simulink model "odev5_tekrar_iremelmas_kara"  (R2023b)
settings: Solver=ode23tb  StartTime=0.0  StopTime=0.1  RelTol=1e-3
libraries: spsCurrentMeasurementLib x18, spsSeriesRLCBranchLib x15, spsMeanLib x9, spsDiodeLib x6, spsMosfetLib x6, spsVoltageMeasurementLib x6, spsDCVoltageSourceLib x3, spsGroundLib x3, spsLinearTransformerLib x3, spsTHDLib x3, spspowerguiLib x1
settings Model: Creator=ireme  LastModifiedBy=ireme

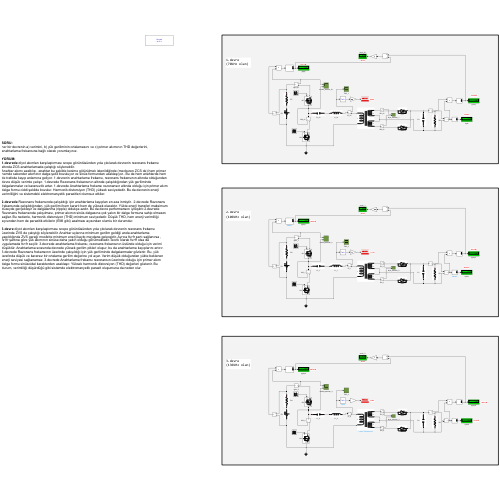
[thumbnail: Simulink's stored preview of the top-level diagram]
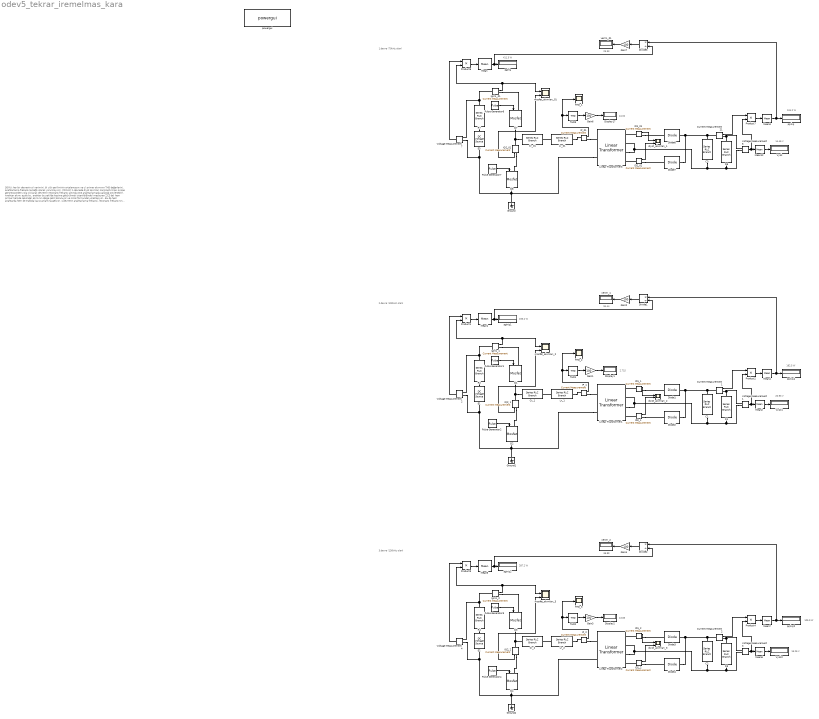
== system odev5_tekrar_iremelmas_kara ==
  note: 1.devre
      | (70kHz olan)
  note: 14.46 V
  note: 2.devre
      | (100kHz olan)
  note: 20.93 V
  note: 3.devre
      | (130kHz olan)
  note: 15.26 V
  note: 104.2 W
  note: 411.3 W
  note: 25.33
  note: 24.02
  note: 182.5 W
  note: 2.715
  note: 94.44
  note: 193.2 W
  note: 105.9 W
  note: 36.89
  note: 13.83
  note: 287.2 W
  note: SORU:
      | her bir devrenin a) verimini, b) yük geriliminin ortalamasını ve c) primer akımının THD değerlerini, anahtarlama frekansına bağlı olarak yorumlayınız.
      |
      | YORUM:
      | 1.devrede diyot akımları karşılaştırması scope görüntüsünden yola çıkılarak devrenin rezonans frekansı altında ZCS anahtarlamada çalıştığı söylenebilir.
      | Anahtar akımı azaltılıp , anahtar bu şekilde kesime götürülmek istenildiğinde (mecburen ZCS de) hem primer hemde sekonder akımının dalga şekli bozuluyor ve sinüs formundan uzaklaşıyor.. Bu da hem anahtarda hem de trafoda kayıp anlamına geliyor. 1.devrenin anahtarlama frekansı, rezonans frekansının altında olduğundan devre düşük verimle çalışır. 1.devrede Rezonans frekansının altında çalışıldığından yük geriliminde dalgalanmalar ve kararsızlık artar. 1.devrede Anahtarlama frekansı rezonansın altında olduğu için primer akım dalga formu ciddi şekilde bozulur. Harmonik distorsiyon (THD) yüksek seviyededir. Bu da devrenin enerji verimliliğini ve sistemdeki elektromanyetik parazitleri olumsuz etkiler.
      |
      | 2.devrede Rezonans frekansında çalışıldığı için anahtarlama kayıpları en aza inmiştir. 2.devrede Rezonans frekansında çalışıldığından, yük gerilimi hem kararlı hem de yüksek olacaktır. Yükte enerji transferi maksimum düzeyde gerçekleşir ve dalgalanma (ripple) oldukça azdır. Bu da devre performansını iyileştirir. 2.devrede Rezonans frekansında çalışılması, primer akımın sinüs dalgasına çok yakın bir dalga formuna sahip olmasını sağlar. Bu nedenle, harmonik distorsiyon (THD) minimum seviyededir. Düşük THD, hem enerji verimliliği açısından hem de parazitik etkilerin (EMI gibi) azalması açısından olumlu bir durumdur.
      |
      | 3.devre diyot akımları karşılaştırması scope görüntüsünden yola çıkılarak devrenin rezonans frekansı üzerinde ZVS de çalıştığı söylenebilir. Anahtar uçlarına minimum gerilim geldiği anda anahtarlama yapıldığında ZVS gereği mosfette minimum enerji kaybı meydana gelecektir. Ayrıca fs>fr şartı sağlanırsa , fs<fr şartına göre yük akımının sinüse daha yakın olduğu görülmektedir.Teorik olarak fs>fr olsa da uygulamada fs<fr seçilir. 3.devrede anahtarlama frekansı, rezonans frekansının üstünde olduğu için verimi düşüktür. Anahtarlama sırasında devrede yüksek gerilim pikleri oluşur, bu da anahtarlama kayıplarını artırır. 3.devrede Rezonans frekansının üzerinde çalışıldığı için yük geriliminde dalgalanmalar gözlenir. Bu, yük tarafında düşük ve kararsız bir ortalama gerilim değerine yol açar. Verim düşük olduğundan yükte beklenen enerji seviyesi sağlanamaz. 3.devrede Anahtarlama frekansı rezonansın üzerinde olduğu için primer akım dalga formu sinüsoidal karakterden uzaklaşır. Yüksek harmonik distorsiyon (THD) değerleri gözlenir. Bu durum, verimliliği düşürdüğü gibi sistemde elektromanyetik parazit oluşumuna da neden olur.
  C1 : spsSeriesRLCBranchLib/Series RLC Branch  LConnTagsString=__new0  RConnTagsString=__new0  BranchType=C  Resistance=1  Inductance=1e-3  SetiL0=off  InitialCurrent=0  Capacitance=150e-3  Setx0=off  InitialVoltage=0  Measurements=None
  C2 : spsSeriesRLCBranchLib/Series RLC Branch  LConnTagsString=__new0  RConnTagsString=__new0  BranchType=C  Resistance=1  Inductance=1e-3  SetiL0=off  InitialCurrent=0  Capacitance=150e-3  Setx0=off  InitialVoltage=0  Measurements=None
  C3 : spsSeriesRLCBranchLib/Series RLC Branch  LConnTagsString=__new0  RConnTagsString=__new0  BranchType=C  Resistance=1  Inductance=1e-3  SetiL0=off  InitialCurrent=0  Capacitance=150e-3  Setx0=off  InitialVoltage=0  Measurements=None
  Cr_01 : spsSeriesRLCBranchLib/Series RLC Branch  LConnTagsString=__new0  RConnTagsString=__new0  BranchType=C  Resistance=1  Inductance=1e-3  SetiL0=off  InitialCurrent=0  Capacitance=22e-9  Setx0=off  InitialVoltage=0  Measurements=None
  Cr_1 : spsSeriesRLCBranchLib/Series RLC Branch  LConnTagsString=__new0  RConnTagsString=__new0  BranchType=C  Resistance=1  Inductance=1e-3  SetiL0=off  InitialCurrent=0  Capacitance=22e-9  Setx0=off  InitialVoltage=0  Measurements=None
  Cr_2 : spsSeriesRLCBranchLib/Series RLC Branch  LConnTagsString=__new0  RConnTagsString=__new0  BranchType=C  Resistance=1  Inductance=1e-3  SetiL0=off  InitialCurrent=0  Capacitance=22e-9  Setx0=off  InitialVoltage=0  Measurements=None
  Current Measurement1 : spsCurrentMeasurementLib/Current Measurement  PhasorSimulation=off  OutputType=Complex  PSBequivalent=0
  Current Measurement2 : spsCurrentMeasurementLib/Current Measurement  PhasorSimulation=off  OutputType=Complex  PSBequivalent=0
  Current Measurement21 : spsCurrentMeasurementLib/Current Measurement  PhasorSimulation=off  OutputType=Complex  PSBequivalent=0
  Diode{1..4,6..7} (6 alike) : spsDiodeLib/Diode  Ron=0.001  Lon=0  Vf=0.8  IC=0  UseSnubber=0  Rs=500  Cs=250e-9  Measurements=off
  Display1 : Display
  Display17 : Display
  Display2 : Display
  Divide1 : Product  Inputs=*/
  Divide2 : Product  Inputs=*/
  Divide3 : Product  Inputs=*/
  E1 : spsDCVoltageSourceLib/DC Voltage Source  Amplitude=390  Measurements=None
  E2 : spsDCVoltageSourceLib/DC Voltage Source  Amplitude=390  Measurements=None
  E3 : spsDCVoltageSourceLib/DC Voltage Source  Amplitude=390  Measurements=None
  Gain{1..4,6..7} (6 alike) : Gain  Gain=100
  Ground : spsGroundLib/Ground  LConnTagsString=a
  Ground1 : spsGroundLib/Ground  LConnTagsString=a
  Ground2 : spsGroundLib/Ground  LConnTagsString=a
  ID1_01 : spsCurrentMeasurementLib/Current Measurement  PhasorSimulation=off  OutputType=Complex  PSBequivalent=0
  ID1_1 : spsCurrentMeasurementLib/Current Measurement  PhasorSimulation=off  OutputType=Complex  PSBequivalent=0
  ID1_2 : spsCurrentMeasurementLib/Current Measurement  PhasorSimulation=off  OutputType=Complex  PSBequivalent=0
  ID2_01 : spsCurrentMeasurementLib/Current Measurement  PhasorSimulation=off  OutputType=Complex  PSBequivalent=0
  ID2_1 : spsCurrentMeasurementLib/Current Measurement  PhasorSimulation=off  OutputType=Complex  PSBequivalent=0
  ID2_2 : spsCurrentMeasurementLib/Current Measurement  PhasorSimulation=off  OutputType=Complex  PSBequivalent=0
  IP_01 : spsCurrentMeasurementLib/Current Measurement  PhasorSimulation=off  OutputType=Complex  PSBequivalent=0
  IP_1 : spsCurrentMeasurementLib/Current Measurement  PhasorSimulation=off  OutputType=Complex  PSBequivalent=0
  IP_2 : spsCurrentMeasurementLib/Current Measurement  PhasorSimulation=off  OutputType=Complex  PSBequivalent=0
  IQ2_01 : spsCurrentMeasurementLib/Current Measurement  PhasorSimulation=off  OutputType=Complex  PSBequivalent=0
  IQ2_1 : spsCurrentMeasurementLib/Current Measurement  PhasorSimulation=off  OutputType=Complex  PSBequivalent=0
  IQ2_2 : spsCurrentMeasurementLib/Current Measurement  PhasorSimulation=off  OutputType=Complex  PSBequivalent=0
  Igiris_01 : spsCurrentMeasurementLib/Current Measurement  PhasorSimulation=off  OutputType=Complex  PSBequivalent=0
  Igiris_1 : spsCurrentMeasurementLib/Current Measurement  PhasorSimulation=off  OutputType=Complex  PSBequivalent=0
  Igiris_2 : spsCurrentMeasurementLib/Current Measurement  PhasorSimulation=off  OutputType=Complex  PSBequivalent=0
  Linear Transformer1 : spsLinearTransformerLib/Linear Transformer  UNITS=SI  NominalPower=[ 300 150e3]  winding1=[36 0 0]  winding2=[4 0 0]  ThreeWindings=on  winding3=[4 0 0]  RmLm=[1e6 565e-06]  Measurements=None  DataType=on
  Linear Transformer2 : spsLinearTransformerLib/Linear Transformer  UNITS=SI  NominalPower=[ 300 150e3]  winding1=[36 0 0]  winding2=[4 0 0]  ThreeWindings=on  winding3=[4 0 0]  RmLm=[1e6 565e-06]  Measurements=None  DataType=on
  Linear Transformer3 : spsLinearTransformerLib/Linear Transformer  UNITS=SI  NominalPower=[ 300 150e3]  winding1=[36 0 0]  winding2=[4 0 0]  ThreeWindings=on  winding3=[4 0 0]  RmLm=[1e6 565e-06]  Measurements=None  DataType=on
  Lr_01 : spsSeriesRLCBranchLib/Series RLC Branch  LConnTagsString=__new0  RConnTagsString=__new0  BranchType=L  Resistance=1  Inductance=113e-6  SetiL0=off  InitialCurrent=0  Capacitance=1e-6  Setx0=off  InitialVoltage=0  Measurements=None
  Lr_1 : spsSeriesRLCBranchLib/Series RLC Branch  LConnTagsString=__new0  RConnTagsString=__new0  BranchType=L  Resistance=1  Inductance=113e-6  SetiL0=off  InitialCurrent=0  Capacitance=1e-6  Setx0=off  InitialVoltage=0  Measurements=None
  Lr_2 : spsSeriesRLCBranchLib/Series RLC Branch  LConnTagsString=__new0  RConnTagsString=__new0  BranchType=L  Resistance=1  Inductance=113e-6  SetiL0=off  InitialCurrent=0  Capacitance=1e-6  Setx0=off  InitialVoltage=0  Measurements=None
  Mean{,1..2,5..6,12} (6 alike) : spsMeanLib/Mean  Freq=50  Vinit=0  Ts=0
  Mean3 : spsMeanLib/Mean  Freq=70e3  Vinit=0  Ts=0
  Mean4 : spsMeanLib/Mean  Freq=100e3  Vinit=0  Ts=0
  Mean7 : spsMeanLib/Mean  Freq=130e3  Vinit=0  Ts=0
  Product{1..4,6..7} (6 alike) : Product
  Pulse Generator1 : DiscretePulseGenerator  PulseType=Time based  Period=1/(100e3)  PulseWidth=50
  Pulse Generator2 : DiscretePulseGenerator  PulseType=Time based  Period=1/(100e3)  PulseWidth=50  PhaseDelay=1/(2*100e3)
  Pulse Generator3 : DiscretePulseGenerator  PulseType=Time based  Period=1/(130e3)  PulseWidth=50
  Pulse Generator4 : DiscretePulseGenerator  PulseType=Time based  Period=1/(130e3)  PulseWidth=50  PhaseDelay=1/(2*130e3)
  Pulse Generator6 : DiscretePulseGenerator  PulseType=Time based  Period=1/(70e3)  PulseWidth=50
  Pulse Generator7 : DiscretePulseGenerator  PulseType=Time based  Period=1/(70e3)  PulseWidth=50  PhaseDelay=1/(2*70e3)
  Q{1..4,7..8} (6 alike) : spsMosfetLib/Mosfet  Ron=0.1  Lon=0  Rd=0.01  Vfd=0  IC=0  Rs=1e5  Cs=inf  Measurements=off
  R1 : spsSeriesRLCBranchLib/Series RLC Branch  LConnTagsString=__new0  RConnTagsString=__new0  BranchType=R  Resistance=2.4  Inductance=1e-3  SetiL0=off  InitialCurrent=0  Capacitance=1e-6  Setx0=off  InitialVoltage=0  Measurements=None
  R2 : spsSeriesRLCBranchLib/Series RLC Branch  LConnTagsString=__new0  RConnTagsString=__new0  BranchType=R  Resistance=1e-6  Inductance=1e-3  SetiL0=off  InitialCurrent=0  Capacitance=1e-6  Setx0=off  InitialVoltage=0  Measurements=None
  R3 : spsSeriesRLCBranchLib/Series RLC Branch  LConnTagsString=__new0  RConnTagsString=__new0  BranchType=R  Resistance=2.4  Inductance=1e-3  SetiL0=off  InitialCurrent=0  Capacitance=1e-6  Setx0=off  InitialVoltage=0  Measurements=None
  R4 : spsSeriesRLCBranchLib/Series RLC Branch  LConnTagsString=__new0  RConnTagsString=__new0  BranchType=R  Resistance=1e-6  Inductance=1e-3  SetiL0=off  InitialCurrent=0  Capacitance=1e-6  Setx0=off  InitialVoltage=0  Measurements=None
  R6 : spsSeriesRLCBranchLib/Series RLC Branch  LConnTagsString=__new0  RConnTagsString=__new0  BranchType=R  Resistance=2.4  Inductance=1e-3  SetiL0=off  InitialCurrent=0  Capacitance=1e-6  Setx0=off  InitialVoltage=0  Measurements=None
  R7 : spsSeriesRLCBranchLib/Series RLC Branch  LConnTagsString=__new0  RConnTagsString=__new0  BranchType=R  Resistance=1e-6  Inductance=1e-3  SetiL0=off  InitialCurrent=0  Capacitance=1e-6  Setx0=off  InitialVoltage=0  Measurements=None
  THD1 : spsTHDLib/THD  Freq=100e3  Ts=0
  THD2 : spsTHDLib/THD  Freq=130e3  Ts=0
  THD3 : spsTHDLib/THD  Freq=70e3  Ts=0
  THD_1 : Scope
  THD_2 : Scope
  THD_3 : Scope
  Voltage Measurement{1..4,6..7} (6 alike) : spsVoltageMeasurementLib/Voltage Measurement  PhasorSimulation=off  OutputType=Complex  PSBequivalent=0
  Vyük : Display
  Vyük1 : Display
  Vyük2 : Display
  diyot_akımları_1 : Scope  NumInputPorts=2
  diyot_akımları_2 : Scope  NumInputPorts=2
  diyot_akımları_3 : Scope  NumInputPorts=2
  mosfet_akımları_01 : Scope  NumInputPorts=2
  mosfet_akımları_2 : Scope  NumInputPorts=2
  mosfet_akımları_3 : Scope  NumInputPorts=2
  pgiriş : Display
  pgiriş1 : Display
  pgiriş2 : Display
  powergui : spspowerguiLib/powergui  Priority=1  SimulationMode=Discrete  SampleTime=1e-7  frequency=60  Iterations=50  frequencyindice=0  Pbase=100e6  ErrMax=1e-4  UnitsV=kV  UnitsW=MW  buscounter=0  FunctionMessages=off  echomessages=off  EnableUseOfTLC=off  CurrentSourceSwitches=off  DisableSnubberDevices=off  DisableRonSwitches=off  DisableVfSwitches=off  DisplayEquations=off  AutomaticDiscreteSolvers=off  SolverType=Tustin/Backward Euler (TBE)  Interpol=off  ExternalGateDelay=off  methode=off  Ts=100  x0status=zero  SPID=on  SwTol=0  HookPort=off  NonlinearTolerance=1e-4  nMaxIteration=100  ContinueOnMaxIteration=off  RestoreLinks=warning  ResistiveCurrentMeasurement=off  Frange=[0:2:500]  Ylog=off  Xlog=on  ShowGrid=off  save=off  variable=ZData  structure=0  ZoomFFT=off  StartTime=0.0  cycles=1  DisplayStyle=1  fundamental=60  FreqAxis=off  MaxFrequency=1000  frequencyindicesteady=1  RmsSteady=1  display=off
  pçıkış : Display
  pçıkış1 : Display
  pçıkış2 : Display
  verim_01 : Display
  verim_1 : Display
  verim_2 : Display
  wires:
  IQ2_01/1 -> mosfet_akımları_01/2
  Pulse Generator7/1 -> Q8/1
  Voltage Measurement6/1 -> Product7/2, Mean12/1
  Voltage Measurement7/1 -> Product6/1
  ID1_01/1 -> diyot_akımları_1/1
  THD3/1 -> Gain6/1
  Gain6/1 -> Display17/1
  Divide3/1 -> Gain7/1
  Gain7/1 -> verim_01/1
  Pulse Generator6/1 -> Q7/1
  Igiris_01/1 -> mosfet_akımları_01/1, Product6/2
  IP_01/1 -> THD_1/1, THD3/1
  ID2_01/1 -> diyot_akımları_1/2
  Mean12/1 -> Vyük/1
  Product6/1 -> Mean/1
  Product7/1 -> Mean3/1
  Mean3/1 -> Divide3/1, pçıkış/1
  Mean/1 -> Divide3/2, pgiriş/1
  Current Measurement21/1 -> Product7/1
  Current Measurement1/1 -> Product2/1
  Mean1/1 -> pgiriş1/1, Divide1/2
  Mean4/1 -> pçıkış1/1, Divide1/1
  Product2/1 -> Mean4/1
  Product1/1 -> Mean1/1
  Mean2/1 -> Vyük1/1
  ID2_1/1 -> diyot_akımları_2/2
  IP_1/1 -> THD1/1, THD_2/1
  Igiris_1/1 -> Product1/2, mosfet_akımları_2/1
  Pulse Generator1/1 -> Q1/1
  Gain2/1 -> verim_1/1
  Divide1/1 -> Gain2/1
  Gain1/1 -> Display1/1
  THD1/1 -> Gain1/1
  ID1_1/1 -> diyot_akımları_2/1
  Voltage Measurement2/1 -> Product1/1
  Voltage Measurement1/1 -> Mean2/1, Product2/2
  Pulse Generator2/1 -> Q2/1
  IQ2_1/1 -> mosfet_akımları_2/2
  IQ2_2/1 -> mosfet_akımları_3/2
  Pulse Generator4/1 -> Q4/1
  Voltage Measurement3/1 -> Product4/2, Mean6/1
  Voltage Measurement4/1 -> Product3/1
  ID1_2/1 -> diyot_akımları_3/1
  THD2/1 -> Gain3/1
  Gain3/1 -> Display2/1
  Divide2/1 -> Gain4/1
  Gain4/1 -> verim_2/1
  Pulse Generator3/1 -> Q3/1
  Igiris_2/1 -> mosfet_akımları_3/1, Product3/2
  IP_2/1 -> THD_3/1, THD2/1
  ID2_2/1 -> diyot_akımları_3/2
  Mean6/1 -> Vyük2/1
  Product3/1 -> Mean5/1
  Product4/1 -> Mean7/1
  Mean7/1 -> Divide2/1, pçıkış2/1
  Mean5/1 -> Divide2/2, pgiriş2/1
  Current Measurement2/1 -> Product4/1
  connections:
  Voltage Measurement6/LConn2 -- R6/RConn1 -- C3/RConn1 -- Linear Transformer3/RConn3 -- Linear Transformer3/RConn2
  C3/LConn1 -- Diode7/RConn1 -- Diode6/RConn1 -- Current Measurement21/LConn1
  Cr_01/LConn1 -- IQ2_01/LConn1 -- Q7/RConn1
  Linear Transformer3/LConn2 -- Ground/LConn1 -- Q8/RConn1 -- Voltage Measurement7/LConn2 -- E3/LConn1
  R7/RConn1 -- E3/RConn1
  Igiris_01/RConn1 -- Q7/LConn1
  ID1_01/LConn1 -- Linear Transformer3/RConn1
  Lr_01/RConn1 -- IP_01/LConn1
  Lr_01/LConn1 -- Cr_01/RConn1
  IQ2_01/RConn1 -- Q8/LConn1
  R7/LConn1 -- Voltage Measurement7/LConn1 -- Igiris_01/LConn1
  ID1_01/RConn1 -- Diode6/LConn1
  IP_01/RConn1 -- Linear Transformer3/LConn1
  ID2_01/RConn1 -- Diode7/LConn1
  ID2_01/LConn1 -- Linear Transformer3/RConn4
  R6/LConn1 -- Current Measurement21/RConn1 -- Voltage Measurement6/LConn1
  Voltage Measurement1/LConn2 -- Linear Transformer1/RConn2 -- Linear Transformer1/RConn3 -- C1/RConn1 -- R1/RConn1
  Diode2/RConn1 -- Diode1/RConn1 -- C1/LConn1 -- Current Measurement1/LConn1
  Cr_1/LConn1 -- Q1/RConn1 -- IQ2_1/LConn1
  Linear Transformer1/LConn2 -- E1/LConn1 -- Voltage Measurement2/LConn2 -- Q2/RConn1 -- Ground1/LConn1
  Voltage Measurement2/LConn1 -- R2/LConn1 -- Igiris_1/LConn1
  Current Measurement1/RConn1 -- R1/LConn1 -- Voltage Measurement1/LConn1
  ID2_1/LConn1 -- Linear Transformer1/RConn4
  ID2_1/RConn1 -- Diode2/LConn1
  IP_1/RConn1 -- Linear Transformer1/LConn1
  ID1_1/RConn1 -- Diode1/LConn1
  IQ2_1/RConn1 -- Q2/LConn1
  Lr_1/LConn1 -- Cr_1/RConn1
  Igiris_1/RConn1 -- Q1/LConn1
  ID1_1/LConn1 -- Linear Transformer1/RConn1
  R2/RConn1 -- E1/RConn1
  Lr_1/RConn1 -- IP_1/LConn1
  Linear Transformer2/RConn2 -- Voltage Measurement3/LConn2 -- R3/RConn1 -- C2/RConn1 -- Linear Transformer2/RConn3
  Diode3/RConn1 -- Current Measurement2/LConn1 -- C2/LConn1 -- Diode4/RConn1
  Q3/RConn1 -- Cr_2/LConn1 -- IQ2_2/LConn1
  E2/LConn1 -- Linear Transformer2/LConn2 -- Ground2/LConn1 -- Q4/RConn1 -- Voltage Measurement4/LConn2
  R4/LConn1 -- Voltage Measurement4/LConn1 -- Igiris_2/LConn1
  R3/LConn1 -- Current Measurement2/RConn1 -- Voltage Measurement3/LConn1
  R4/RConn1 -- E2/RConn1
  ID1_2/LConn1 -- Linear Transformer2/RConn1
  Igiris_2/RConn1 -- Q3/LConn1
  Lr_2/LConn1 -- Cr_2/RConn1
  IQ2_2/RConn1 -- Q4/LConn1
  ID2_2/LConn1 -- Linear Transformer2/RConn4
  ID2_2/RConn1 -- Diode4/LConn1
  Lr_2/RConn1 -- IP_2/LConn1
  ID1_2/RConn1 -- Diode3/LConn1
  IP_2/RConn1 -- Linear Transformer2/LConn1
